simulink library "FirGenericDeprecated"  (R2022b)
settings: Solver=VariableStepAuto  StartTime=0.0  StopTime=10.0  RelTol=1e-3
libraries: HandyTextFile x7, FeaturePath x1, ITC x1
settings Model: Creator=fz1054048  LastModifiedBy=fz1054048

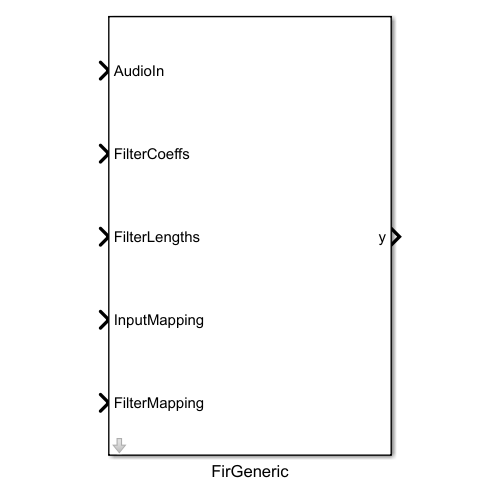
[thumbnail: Simulink's stored preview of the top-level diagram]
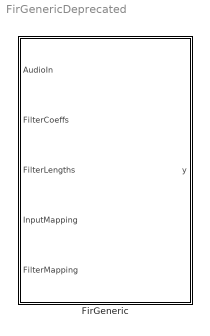
== system FirGenericDeprecated ==
  FirGeneric : Subsystem  mask(FirGeneric){Config=[]}
      mask prompts: Config "FirGenericConfig"
      mask help:
      | FirGeneric is a configurable multi-channel FIR filter that supports one or more channels.  Different filter coefficients and number of coefficients can be used for each channel filter.  There can be fewer inputs than outputs, with some inputs routed to more than one output filter. Identical filter configurations can also be used for multiple output filters. FirGeneric supports multiple hardware implementations.
      |
      | For more information, see 'Help'.
      mask init:
      | blkh=gcbh;
      | Config=BTConfig.Assert(blkh,Config);
      | 
      | Config.Validate();
      | Config.DoMaskInit(blkh);
      mask Help:
      | Generic multi-channel FIR block supports multiple inputs, outputs and coefficient sets. Some inputs may drive multiple outputs, and this input sharing is specified by an input mapping per output. Some filters may be shared among multiple outputs, and this filter sharing is specified by a filter mapping per output. Input sharing assumes all filters sharing the same input have the same length to support state buffer sharing.
      | 
      | Input signals:
      | AudioIn: input channels [frame size x number of inputs]
      | FilterCoeffs: coefficient sets [total sum of filter lengths x 1]
      | FilterLengths: array of filter lengths [number of filters x 1]
      | InputMapping: zero-based input mapping for each output [number of outputs x 1]
      | FilterMapping:  zero-based filter mapping for each output [number of outputs x 1]
      | 
      | Output signals:
      | y: output channels [frame size x number of outputs]
      | 
      | 
      | For Sharc: The FirGeneric CodeWorkMemory buffer should always be mapped to L1 memory or core MIPS usage will increase.
      | For Hexagon: The filter lengths for each channel must be a multiple of 4.

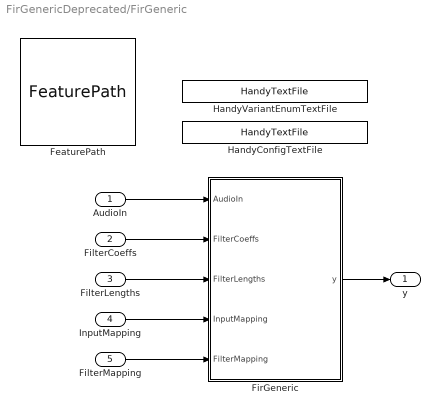
== system FirGenericDeprecated/FirGeneric ==
  AudioIn : Inport
  FilterCoeffs : Inport  Port=2
  FilterLengths : Inport  Port=3
  InputMapping : Inport  Port=4
  FilterMapping : Inport  Port=5
  FeaturePath : FeaturePath/FeaturePath  FeatureName=FIR  IsGroup=off  GroupNumber=-1  IsModule=off  TriggerInit=[-5 -21 110 86]
      settings: SourceProductName=Bose Talaria
  FirGeneric : Subsystem  Variant=on
  HandyConfigTextFile : HandyTextFile/HandyTextFile  TemplateSource=Config  FileSuffix=File  OpenDialogOnLoad=off  UseThisBlockName=off  AddGrandParentNamePrefix=off  TheDefaultText=% $(FILENAME) $(PREFIX) $(SUFFIX)  ShowInLibBrowser=on
      settings: SourceProductName=Bose Talaria
  HandyVariantEnumTextFile : HandyTextFile/HandyTextFile  TemplateSource=VariantEnum  FileSuffix=File  OpenDialogOnLoad=off  UseThisBlockName=off  AddGrandParentNamePrefix=off  TheDefaultText=% $(FILENAME) $(PREFIX) $(SUFFIX)  ShowInLibBrowser=on
      settings: SourceProductName=Bose Talaria
  y : Outport
  wires:
  AudioIn/1 -> FirGeneric/1(AudioIn)
  FilterCoeffs/1 -> FirGeneric/2(FilterCoeffs)
  FilterLengths/1 -> FirGeneric/3(FilterLengths)
  InputMapping/1 -> FirGeneric/4(InputMapping)
  FilterMapping/1 -> FirGeneric/5(FilterMapping)
  FirGeneric/1(y) -> y/1

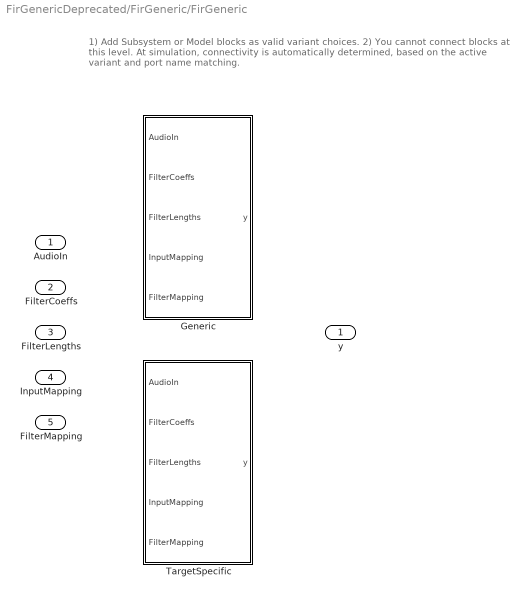
== system FirGenericDeprecated/FirGeneric/FirGeneric ==
  note: 1) Add Subsystem or Model blocks as valid variant choices.
      | 2) You cannot connect blocks at this level. At simulation, connectivity is automatically
      | determined, based on the active variant and port name matching.
  AudioIn : Inport
  FilterCoeffs : Inport  Port=2
  FilterLengths : Inport  Port=3
  InputMapping : Inport  Port=4
  FilterMapping : Inport  Port=5
  Generic : Subsystem  VariantControl=(default)
  TargetSpecific : Subsystem  VariantControl="(Config.Variant.StartsWith(\"Sharc\")) || (Config.Variant == \"Hexagon\") || (Config.Variant == \"ArmNeonV7V8\")"
  y : Outport

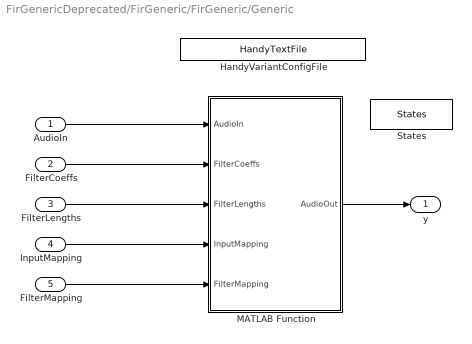
== system FirGenericDeprecated/FirGeneric/FirGeneric/Generic ==
  AudioIn : Inport
  FilterCoeffs : Inport  Port=2
  FilterLengths : Inport  Port=3
  InputMapping : Inport  Port=4
  FilterMapping : Inport  Port=5
  HandyVariantConfigFile : HandyTextFile/HandyTextFile  TemplateSource=VariantConfig  FileSuffix=Init  OpenDialogOnLoad=off  UseThisBlockName=off  AddGrandParentNamePrefix=on  TheDefaultText=|  ShowInLibBrowser=on
      | % $(FILENAME) Setup model parameters for each "Init" callback (e.g. update diagram)
      | sample_rate_in_hertz = 44100;
      | frame_size = 32;
      | sysin_channel_count = 2;
      settings: SourceProductName=Bose Talaria
  MATLAB Function : MATLAB Function  TreatAsAtomicUnit=on  mask{FrameSize=Config.FrameSize, NumInputs=Config.NumInputs, NumOutputs=Config.NumOutputs, StateBufferSize=Config.VariantObj.StateBufferSize}
  States : DataStoreMemory  DataStoreName=States  WriteAfterWriteMsg=warning  InitialValue=single(zeros(Config.VariantObj.StateBufferSize,1))  ShowAdditionalParam=off  OutDataTypeStr=single
  y : Outport
  wires:
  AudioIn/1 -> MATLAB Function/1(AudioIn)
  FilterCoeffs/1 -> MATLAB Function/2(FilterCoeffs)
  FilterLengths/1 -> MATLAB Function/3(FilterLengths)
  InputMapping/1 -> MATLAB Function/4(InputMapping)
  FilterMapping/1 -> MATLAB Function/5(FilterMapping)
  MATLAB Function/1(AudioOut) -> y/1

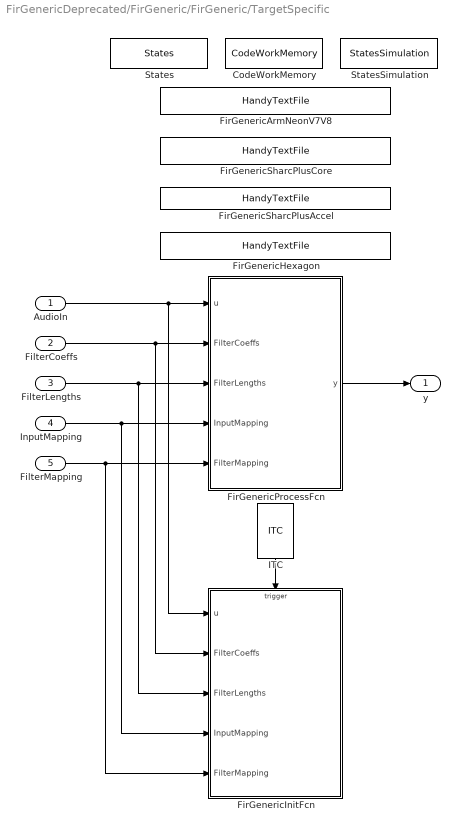
== system FirGenericDeprecated/FirGeneric/FirGeneric/TargetSpecific ==
  AudioIn : Inport
  FilterCoeffs : Inport  Port=2
  FilterLengths : Inport  Port=3
  InputMapping : Inport  Port=4
  FilterMapping : Inport  Port=5
  CodeWorkMemory : DataStoreMemory  DataStoreName=CodeWorkMemory  WriteAfterWriteMsg=warning  InitialValue=uint32(zeros(1,Config.VariantObj.CodeWorkMemorySize))  ShowAdditionalParam=off  OutDataTypeStr=uint32
  FirGenericArmNeonV7V8 : HandyTextFile/HandyTextFile  TemplateSource=VariantConfig  FileSuffix=Init  OpenDialogOnLoad=off  UseThisBlockName=on  AddGrandParentNamePrefix=off  TheDefaultText=|  ShowInLibBrowser=on
      | % $(FILENAME) Setup model parameters for each "Init" callback (e.g. update diagram)
      | sample_rate_in_hertz = 44100;
      | frame_size = 32;
      | sysin_channel_count = 2;
      settings: SourceProductName=Bose Talaria
  FirGenericHexagon : HandyTextFile/HandyTextFile  TemplateSource=VariantConfig  FileSuffix=Init  OpenDialogOnLoad=off  UseThisBlockName=on  AddGrandParentNamePrefix=off  TheDefaultText=|  ShowInLibBrowser=on
      | % $(FILENAME) Setup model parameters for each "Init" callback (e.g. update diagram)
      | sample_rate_in_hertz = 44100;
      | frame_size = 32;
      | sysin_channel_count = 2;
      settings: SourceProductName=Bose Talaria
  FirGenericInitFcn : MATLAB Function  TreatAsAtomicUnit=on  mask{VariantUint8=Config.Variant.Uint8Str}
  FirGenericProcessFcn : MATLAB Function  TreatAsAtomicUnit=on  mask{VariantUint8=Config.Variant.Uint8Str}
  FirGenericSharcPlusAccel : HandyTextFile/HandyTextFile  TemplateSource=VariantConfig  FileSuffix=Init  OpenDialogOnLoad=off  UseThisBlockName=on  AddGrandParentNamePrefix=off  TheDefaultText=|  ShowInLibBrowser=on
      | % $(FILENAME) Setup model parameters for each "Init" callback (e.g. update diagram)
      | sample_rate_in_hertz = 44100;
      | frame_size = 32;
      | sysin_channel_count = 2;
      settings: SourceProductName=Bose Talaria
  FirGenericSharcPlusCore : HandyTextFile/HandyTextFile  TemplateSource=VariantConfig  FileSuffix=Init  OpenDialogOnLoad=off  UseThisBlockName=on  AddGrandParentNamePrefix=off  TheDefaultText=|  ShowInLibBrowser=on
      | % $(FILENAME) Setup model parameters for each "Init" callback (e.g. update diagram)
      | sample_rate_in_hertz = 44100;
      | frame_size = 32;
      | sysin_channel_count = 2;
      settings: SourceProductName=Bose Talaria
  ITC : ITC/ITC
      settings: SourceProductName=Bose Talaria
  States : DataStoreMemory  DataStoreName=States  WriteAfterWriteMsg=warning  InitialValue=single(zeros(Config.VariantObj.StateBufferSize,1))  ShowAdditionalParam=off  OutDataTypeStr=single
  StatesSimulation : DataStoreMemory  DataStoreName=StatesSimulation  WriteAfterWriteMsg=warning  InitialValue=single(zeros(Config.StateBufferSizeSimulation,1))  ShowAdditionalParam=off  OutDataTypeStr=single
  y : Outport
  wires:
  FirGenericProcessFcn/1(y) -> y/1
  FilterMapping/1 -> FirGenericInitFcn/5(FilterMapping), FirGenericProcessFcn/5(FilterMapping)
  InputMapping/1 -> FirGenericInitFcn/4(InputMapping), FirGenericProcessFcn/4(InputMapping)
  FilterLengths/1 -> FirGenericInitFcn/3(FilterLengths), FirGenericProcessFcn/3(FilterLengths)
  FilterCoeffs/1 -> FirGenericInitFcn/2(FilterCoeffs), FirGenericProcessFcn/2(FilterCoeffs)
  AudioIn/1 -> FirGenericInitFcn/1(u), FirGenericProcessFcn/1(u)
  ITC/1 -> FirGenericInitFcn/Trigger

== matlab function FirGenericDeprecated/FirGeneric/FirGeneric/TargetSpecific/FirGenericProcessFcn ==
  data: u input; y output; FilterCoeffs input; FilterLengths input; InputMapping input; FilterMapping input; VariantUint8 parameter; States data_store_memory; CodeWorkMemory data_store_memory; StatesSimulation data_store_memory
function y = FirGenericProcess(u, FilterCoeffs, FilterLengths, InputMapping, FilterMapping, VariantUint8)
% Generic FIR function to work with M inputs, N outputs and K filters
%
% Parameters:
%   u:              input channels [frame size x number of inputs]
%   FilterCoeffs:   coefficient sets [total filter lengths x 1]
%   FilterLengths:  array of filter lengths [number of filters x 1]
%   InputMapping:   zero-based input mapping for each filter  [number of outputs x 1]
%   FilterMapping:  zero-based filter mapping for each filter [number of outputs x 1]
%   VariantStr:     string corresponding to the variant type
%
% Global parameters:
%   States:         array of states [totalBufferSize x 1]
%   CodeWorkMemory: working memory set up during roommode reset/init CRL
%                   function call [codeWorkMemorySize x 1]
%--------------------------------------------------------------------------


% Extract configuration information from inputs
[FrameSize, NumInputs]  = size(u);
NumOutputs = numel(InputMapping);

global States;
global CodeWorkMemory;
global StatesSimulation

% Define persistent variables for SharcPlusAccel Variant
persistent DelayedOut;
    
% Set correct data types
FilterLengths = uint32(FilterLengths);
FrameSize = uint32(FrameSize);
NumOutputs = uint32(NumOutputs);
InputMapping = uint32(InputMapping);

% Reconstitute Variant
VariantSelect = char(VariantUint8);

% Simulation
if(coder.target('MATLAB') || coder.target('Sfun')) 
    switch(VariantSelect)
        case {'SharcPlusAccel'}
            % Define one-frame delay buffer only for Accelerator simulation 
            % Simulink will optimize this out for code generation
            if isempty(DelayedOut)
                DelayedOut = single(zeros(FrameSize, NumOutputs));
            end
            % Manually insert one-frame delay in simulation to mimic 
            % Accelerator behavior
            y = DelayedOut;
            DelayedOut = FirGenericProcessSim(u, FilterCoeffs, numel(StatesSimulation), FilterLengths, InputMapping, ...
                FilterMapping, FrameSize, NumOutputs, VariantSelect);
        otherwise
            y = FirGenericProcessSim(u, FilterCoeffs, numel(StatesSimulation), FilterLengths, InputMapping, ...
                FilterMapping, FrameSize, NumOutputs, VariantSelect);

    end
% Code Generation: same function prototype for core and accel
else
    switch(VariantSelect)

        case {'SharcPlusCore'}
            y = fir_core_process(u, CodeWorkMemory, NumOutputs);
        case {'SharcPlusAccel'}
            y = fir_accelerator_process(u, CodeWorkMemory, NumOutputs);
        case {'Hexagon'}
            y = fir_hexagon_process(u, CodeWorkMemory, NumOutputs);
        case {'ArmNeonV7V8'}
            y = fir_armv7v8_process(single(u), uint32(CodeWorkMemory), uint32(NumOutputs));
    
    end

end

end



%% CRL functions for code generation
function y = fir_core_process(u, WorkMemory, NumOutputs)
% If target == codegen, error out if no CRL found
coder.replace('-errorifnoreplacement');
[FrameSize, ~]  = size(u);
y = single(zeros(FrameSize, NumOutputs));
end

function y = fir_accelerator_process(u, WorkMemory, NumOutputs)
% If target == codegen, error out if no CRL found
coder.replace('-errorifnoreplacement');
[FrameSize, ~]  = size(u);
y = single(zeros(FrameSize, NumOutputs));
end

function y = fir_hexagon_process(u, workMemory, numOutputs)
% If target == codegen, error out if no CRL found
coder.replace('-errorifnoreplacement');
[frameSize, ~]  = size(u);
y = single(zeros(frameSize, numOutputs));
end

function y = fir_armv7v8_process(u, workMemory, numOutputs)
% If target == codegen, error out if no CRL found
coder.replace('-errorifnoreplacement');
[frameSize, ~]  = size(u);
y = single(zeros(frameSize, numOutputs));
end

== matlab function FirGenericDeprecated/FirGeneric/FirGeneric/Generic/MATLAB Function ==
  data: AudioIn input; AudioOut output; FilterCoeffs input; FilterLengths input; InputMapping input; FilterMapping input; NumInputs parameter; FrameSize parameter; NumOutputs parameter; StateBufferSize parameter; States data_store_memory
function AudioOut = FirGenericProcess(AudioIn, FilterCoeffs, FilterLengths, InputMapping, FilterMapping, NumInputs, FrameSize, NumOutputs, StateBufferSize)
global States;
AudioOut = FirGenericProcessSim(AudioIn, FilterCoeffs, numel(States), FilterLengths, ...
                InputMapping, FilterMapping, FrameSize, NumOutputs);

end

== matlab function FirGenericDeprecated/FirGeneric/FirGeneric/TargetSpecific/FirGenericInitFcn ==
  data: u input; FilterCoeffs input; FilterLengths input; InputMapping input; FilterMapping input; VariantUint8 parameter; States data_store_memory; CodeWorkMemory data_store_memory
  events: trigger input FUNCTION_CALL_EVENT
 function FirGenericInit(u, FilterCoeffs, FilterLengths, InputMapping, FilterMapping, VariantUint8)
% Generic FIR function to work with M inputs, N outputs and K filters
%
% Parameters:
%   u:              input channels [frame size x number of inputs]
%   Filteroeffs:    coefficient sets [total filter lengths x 1]
%   FilterLengths:  array of filter lengths [number of filters x 1]
%   InputMapping:   zero-based input mapping for each filter  [number of outputs x 1]
%   FilterMapping:  zero-based filter mapping for each filter [number of outputs x 1]
%
% Global parameters:
%   States:         array of states [totalBufferSize x 1]
%   CodeWorkMemory: working memory set up during roommode reset/init CRL
%                   function call [codeWorkMemorySize x 1]
%--------------------------------------------------------------------------

% Extract configuration information from inputs
[FrameSize, NumInputs]  = size(u);
NumOutputs = numel(InputMapping);

global States;
global CodeWorkMemory;

% Get the work memory and states size
WorkMemorySize = numel(CodeWorkMemory);
StatesSize = numel(States);

% Set correct data types
FilterLengths = uint32(FilterLengths);
NumCoeffSets = uint32(numel(FilterLengths));
FrameSize = uint32(FrameSize);
NumOutputs = uint32(NumOutputs);
NumInputs = uint32(NumInputs);
WorkMemorySize = uint32(WorkMemorySize);
StatesSize = uint32(StatesSize);

% Reconstitute Variant
VariantSelect = char(VariantUint8);

switch(VariantSelect)
    case {'SharcPlusCore'}
        y = fir_core_init(u, FilterCoeffs, States, FilterLengths, InputMapping, FilterMapping, ...
            FrameSize, NumCoeffSets, NumInputs, NumOutputs, CodeWorkMemory);
        CodeWorkMemory(1) = y;
        
    case {'SharcPlusAccel'}
        y = fir_accelerator_init(u, FilterCoeffs, States, StatesSize, FilterLengths, InputMapping, ...
            FilterMapping, FrameSize, NumCoeffSets, NumInputs, NumOutputs, ...
            CodeWorkMemory, WorkMemorySize);
        CodeWorkMemory(1) = y;

    case {'Hexagon'}
        y = fir_hexagon_init(u, FilterCoeffs, States, FilterLengths, InputMapping, FilterMapping, ...
            FrameSize, NumCoeffSets, NumInputs, NumOutputs, CodeWorkMemory);
        CodeWorkMemory(1) = y;
    case {'ArmNeonV7V8'}
        y = fir_armv7v8_init(u, FilterCoeffs, States, FilterLengths, InputMapping, FilterMapping, ...
            FrameSize, NumCoeffSets, NumInputs, NumOutputs, CodeWorkMemory);
        CodeWorkMemory(1) = y;
end

end


function y = fir_accelerator_init(u, coeffs, states, statesSize, filterLengths, inputMapping, filterMapping,...
                                  frameSize, numCoeffSets, numInputs, numOutputs, workMemory,...
                                  workMemorySize)                         
% If target == codegen, error out if no CRL found
coder.replace('-errorifnoreplacement');

% No init simulation code, but need to do something to ensure CRL does not
% get optimized out
y = workMemory(1) + 1;

end

function y = fir_core_init(u, coeffs, states, filterLengths, inputMapping, filterMapping,...
                             frameSize, numCoeffSets, numInputs, numOutputs, workMemory)
% If target == codegen, error out if no CRL found
coder.replace('-errorifnoreplacement');

% No init simulation code, but need to do something to ensure CRL does not
% get optimized out
y = workMemory(1) + 1;

end


function y = fir_hexagon_init(u, coeffs, states, filterLengths, inputMapping, filterMapping,...
                             frameSize, numCoeffSets, numInputs, numOutputs, workMemory)
% If target == codegen, error out if no CRL found
coder.replace('-errorifnoreplacement');

% No init simulation code, but need to do something to ensure CRL does not
% get optimized out
y = workMemory(1) + 1;

end

function y = fir_armv7v8_init(u, coeffs, states, filterLengths, inputMapping, filterMapping,...
                             frameSize, numCoeffSets, numInputs, numOutputs, workMemory)
% If target == codegen, error out if no CRL found
coder.replace('-errorifnoreplacement');

% No init simulation code, but need to do something to ensure CRL does not
% get optimized out
y = workMemory(1) + 1;

end
